simulink model "soal1ghesmateba"  (R2019b)
settings: Solver=VariableStepAuto  StartTime=0.0  StopTime=10  RelTol=1e-3
libraries: simulink x1
settings Model: Creator=user  LastModifiedBy=user

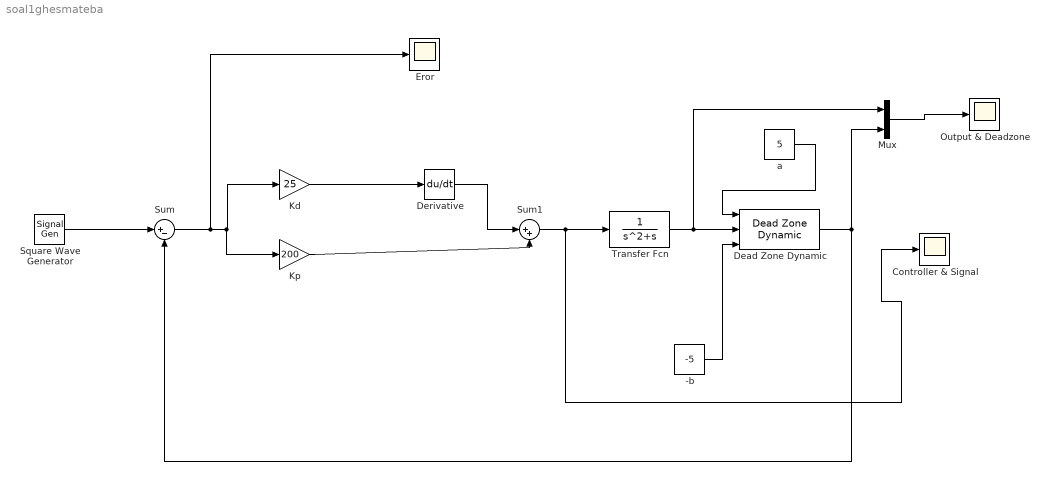
== system soal1ghesmateba ==
  -b : Constant  Value=-5
  Controller & Signal : Scope
  Dead Zone Dynamic : simulink/Discontinuities/Dead Zone Dynamic
      settings: SourceProductName=Simulink  SourceProductBaseCode=SL
  Derivative : Derivative
  "Eror " : Scope
  "Kd " : Gain  Gain=25
  Kp : Gain  Gain=200
  Mux : Mux  Inputs=2
  "Output & Deadzone " : Scope
  "Square Wave Generator " : SignalGenerator  WaveForm=square  Amplitude=10  Frequency=2.5  Units=rad/sec
  Sum : Sum  Inputs=|+-
  Sum1 : Sum  Inputs=|++
  Transfer Fcn : TransferFcn  Denominator=[1 1 0]
  a : Constant  Value=5
  wires:
  Kp/1 -> Sum1/2
  Sum/1 -> "Eror "/1, "Kd "/1, Kp/1
  "Square Wave Generator "/1 -> Sum/1
  Sum1/1 -> Controller & Signal/1, Transfer Fcn/1
  Transfer Fcn/1 -> Mux/1, Dead Zone Dynamic/2
  Derivative/1 -> Sum1/1
  "Kd "/1 -> Derivative/1
  a/1 -> Dead Zone Dynamic/1
  -b/1 -> Dead Zone Dynamic/3
  Mux/1 -> "Output & Deadzone "/1
  Dead Zone Dynamic/1 -> Mux/2, Sum/2
